simulink model "DCMG_model02"  (R2023a)
settings: Solver=FixedStepDiscrete  StartTime=0.0  StopTime=7  FixedStep=Ts  RelTol=1e-3
InitFcn:
  | Ts=10e-6;
  | R1=0.5;
  | R2=0.6;
  | RD1=4;
  | RD2=4;
  | Vdc1=350;
  | Vdc2=350;
  | Vdcmg_ref=125;
  | Vc1_ref=125;
  | Vc2_ref=125;
libraries: spsSeriesRLCBranchLib x7, spsCurrentMeasurementLib x5, slpidlib x5, spsVoltageMeasurementLib x3, spsDiodeLib x3, spsMosfetLib x3, spsControlledCurrentSourceLib x2, spsDCVoltageSourceLib x2, spsGroundLib x1, spsThreePhaseBreakerLib x1, sps_lib x1
settings Model: Creator=Aminsystem  LastModifiedBy=Aminsystem
settings DataIOCC: SaveOutput=off  SignalLogging=off  DSMLogging=off  SaveTime=off  ReturnWorkspaceOutputs=off

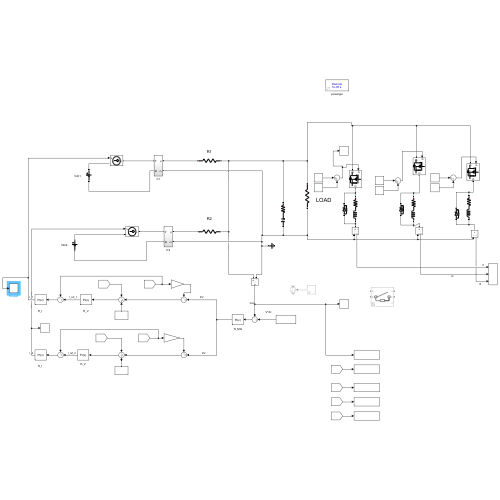
[thumbnail: Simulink's stored preview of the top-level diagram]
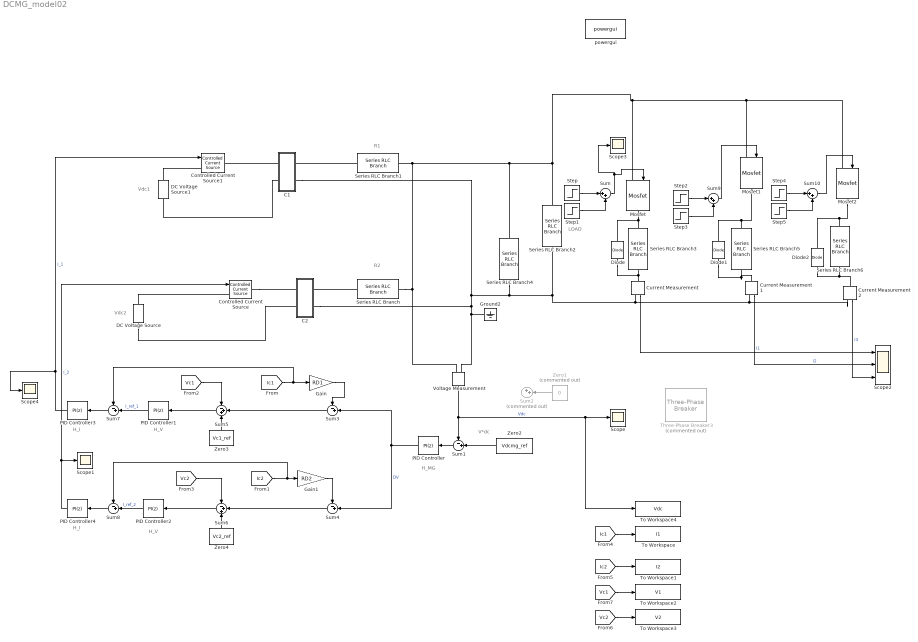
== system DCMG_model02 ==
  note: H_V
  note: Vdc2
  note: Vdc1
  note: R2
  note: V*dc
  note: LOAD
  note: R1
  note: H_V
  note: H_MG
  note: H_I
  note: H_I
  C1 : Subsystem
  C2 : Subsystem
  Controlled Current Source : spsControlledCurrentSourceLib/Controlled Current Source  Initialize=on  Source_Type=DC  Amplitude=0  Phase=0  Frequency=0  Measurements=None
  Controlled Current Source1 : spsControlledCurrentSourceLib/Controlled Current Source  Initialize=on  Source_Type=DC  Amplitude=0  Phase=0  Frequency=0  Measurements=None
  Current Measurement : spsCurrentMeasurementLib/Current Measurement  PhasorSimulation=off  OutputType=Complex  PSBequivalent=0
  Current Measurement1 : spsCurrentMeasurementLib/Current Measurement  PhasorSimulation=off  OutputType=Complex  PSBequivalent=0
  Current Measurement2 : spsCurrentMeasurementLib/Current Measurement  PhasorSimulation=off  OutputType=Complex  PSBequivalent=0
  DC Voltage Source : spsDCVoltageSourceLib/DC Voltage Source  Amplitude=Vdc2  Measurements=None
  DC Voltage Source1 : spsDCVoltageSourceLib/DC Voltage Source  Amplitude=Vdc1  Measurements=None
  Diode : spsDiodeLib/Diode  Ron=0.001  Lon=0  Vf=0.8  IC=0  UseSnubber=0  Rs=500  Cs=250e-9  Measurements=off
  Diode1 : spsDiodeLib/Diode  Ron=0.001  Lon=0  Vf=0.8  IC=0  UseSnubber=0  Rs=500  Cs=250e-9  Measurements=off
  Diode2 : spsDiodeLib/Diode  Ron=0.001  Lon=0  Vf=0.8  IC=0  UseSnubber=0  Rs=500  Cs=250e-9  Measurements=off
  Gain : Gain  Gain=RD1
  Gain1 : Gain  Gain=RD2
  Ground2 : spsGroundLib/Ground  LConnTagsString=a
  Mosfet : spsMosfetLib/Mosfet  Ron=0.1  Lon=0  Rd=0.01  Vfd=0  IC=0  Rs=1e5  Cs=inf  Measurements=off
  Mosfet1 : spsMosfetLib/Mosfet  Ron=0.1  Lon=0  Rd=0.01  Vfd=0  IC=0  Rs=1e5  Cs=inf  Measurements=off
  Mosfet2 : spsMosfetLib/Mosfet  Ron=0.1  Lon=0  Rd=0.01  Vfd=0  IC=0  Rs=1e5  Cs=inf  Measurements=off
  PID Controller{,1..4} (5 alike) : slpidlib/PID Controller  Controller=PI  Form=Parallel  TimeDomain=Discrete-time  UseExternalTs=off  SampleTime=Ts  IntegratorMethod=Forward Euler  FilterMethod=Forward Euler  ControllerParametersSource=internal  P=10  I=100  UseKiTs=off  D=0  N=100  UseFilter=on  TunerSelectOption=Transfer Function Based (PID Tuner App)  InitialConditionSource=internal  InitialConditionForIntegrator=0  InitialConditionForFilter=0  DifferentiatorICPrevScaledInput=0  ExternalReset=none  TrackingMode=off  Kt=1  LimitOutput=off  SatLimitsSource=internal  UpperSaturationLimit=inf  LowerSaturationLimit=-inf  LinearizeAsGain=on  AntiWindupMode=none  Kb=1  LimitIntegrator=off  UpperIntegratorSaturationLimit=inf  LowerIntegratorSaturationLimit=-inf  POutMin=[]  POutMax=[]  IOutMin=[]  IOutMax=[]  DOutMin=[]  DOutMax=[]  NOutMin=[]  NOutMax=[]  SumOutMin=[]  SumOutMax=[]  SaturationOutMin=[]  SaturationOutMax=[]  PParamMin=[]  PParamMax=[]  IParamMin=[]  IParamMax=[]  DParamMin=[]  DParamMax=[]  NParamMin=[]  NParamMax=[]  KbParamMin=[]  KbParamMax=[]  KtParamMin=[]  KtParamMax=[]  KbOutMin=[]  KbOutMax=[]  KtOutMin=[]  KtOutMax=[]  IntegratorOutMin=[]  IntegratorOutMax=[]  FilterOutMin=[]  FilterOutMax=[]  SumI1OutMin=[]  SumI1OutMax=[]  SumI2OutMin=[]  SumI2OutMax=[]  SumI3OutMin=[]  SumI3OutMax=[]  SumI4OutMin=[]  SumI4OutMax=[]  SumDOutMin=[]  SumDOutMax=[]  DifferentiatorOutMin=[]  DifferentiatorOutMax=[]  FilterDiffOutCoefMin=[]  FilterDiffOutCoefMax=[]  ReciprocalOutMin=[]  ReciprocalOutMax=[]  SumDenOutMin=[]  SumDenOutMax=[]  SumNumOutMin=[]  SumNumOutMax=[]  DivideOutMin=[]  DivideOutMax=[]  UdiffTsProdOutMin=[]  UdiffTsProdOutMax=[]  NTsProdOutMin=[]  NTsProdOutMax=[]  UintegralTsProdOutMin=[]  UintegralTsProdOutMax=[]  UngainTsProdOutMin=[]  UngainTsProdOutMax=[]  ClampingZeroOutDataTypeStr=Inherit: Inherit via back propagation  ClampingZeroOutMin=[]  ClampingZeroOutMax=[]  FilterDenConstantOutDataTypeStr=Inherit: Inherit via back propagation  FilterDenConstantOutMin=[]  FilterDenConstantOutMax=[]  PCopyOutDataTypeStr=Inherit: Inherit via back propagation  PCopyOutMin=[]  PCopyOutMax=[]  NCopyOutDataTypeStr=Inherit: Inherit via back propagation  NCopyOutMin=[]  NCopyOutMax=[]  IntegratorContinuousStateAttributes=''  IntegratorStateMustResolveToSignalObject=off  IntegratorRTWStateStorageClass=Auto  FilterContinuousStateAttributes=''  FilterStateMustResolveToSignalObject=off  FilterRTWStateStorageClass=Auto  ParallelPVariant=InternalParameters  IdealPVariant=Disabled  IVariant=InternalParameters  DVariant=Disabled  IntegratorVariant=Discrete  SatVariant=Disabled  AWVariant=Passthrough  PCopyVariant=Disabled  TRVariant=Disabled  FdbkBlocksVariant=Forward  IdealPFdbkVariant=Disabled  SatFdbkVariant=Disabled  DerivativeFilterVariant=Disabled  NVariant=Disabled  NCopyVariant=Disabled_SignalSpec  FilterICVariant=Disabled  IntegratorICVariant=InternalICs  ExternalResetVariant=Disabled  TRSumVariant=Passthrough  SumFdbkVariant=Disabled  SumVariant=Sum_PI  TsampFilterVariant=InternalTs  TsampNgainVariant=Passthrough  TsampIntegralVariant=Disabled_SignalSpec  ExternalSaturationOutDataTypeStr=Inherit: Same as second input
  Scope{,1,3..4} (4 alike) : Scope
  Scope2 : Scope  NumInputPorts=3
  Series RLC Branch : spsSeriesRLCBranchLib/Series RLC Branch  LConnTagsString=__new0  RConnTagsString=__new0  BranchType=R  Resistance=R2  Inductance=1e-3  SetiL0=off  InitialCurrent=0  Capacitance=1e-6  Setx0=off  InitialVoltage=0  Measurements=None
  Series RLC Branch1 : spsSeriesRLCBranchLib/Series RLC Branch  LConnTagsString=__new0  RConnTagsString=__new0  BranchType=R  Resistance=R1  Inductance=1e-3  SetiL0=off  InitialCurrent=0  Capacitance=1e-6  Setx0=off  InitialVoltage=0  Measurements=None
  Series RLC Branch2 : spsSeriesRLCBranchLib/Series RLC Branch  LConnTagsString=__new0  RConnTagsString=__new0  BranchType=R  Resistance=120  Inductance=1e-3  SetiL0=off  InitialCurrent=0  Capacitance=1e-6  Setx0=off  InitialVoltage=0  Measurements=None
  Series RLC Branch3 : spsSeriesRLCBranchLib/Series RLC Branch  LConnTagsString=__new0  RConnTagsString=__new0  BranchType=RL  Resistance=1  Inductance=2e-3  SetiL0=off  InitialCurrent=0  Capacitance=1e-6  Setx0=off  InitialVoltage=0  Measurements=None
  Series RLC Branch4 : spsSeriesRLCBranchLib/Series RLC Branch  LConnTagsString=__new0  RConnTagsString=__new0  BranchType=RC  Resistance=0.1  Inductance=1e-3  SetiL0=off  InitialCurrent=0  Capacitance=100e-6  Setx0=on  InitialVoltage=80  Measurements=None
  Series RLC Branch5 : spsSeriesRLCBranchLib/Series RLC Branch  LConnTagsString=__new0  RConnTagsString=__new0  BranchType=RL  Resistance=0.5  Inductance=5e-3  SetiL0=off  InitialCurrent=0  Capacitance=1e-6  Setx0=off  InitialVoltage=0  Measurements=None
  Series RLC Branch6 : spsSeriesRLCBranchLib/Series RLC Branch  LConnTagsString=__new0  RConnTagsString=__new0  BranchType=RL  Resistance=1  Inductance=10e-3  SetiL0=off  InitialCurrent=0  Capacitance=1e-6  Setx0=off  InitialVoltage=0  Measurements=None
  Step : Step  Time=1.3  SampleTime=Ts
  Step1 : Step  Time=2.3  After=-1  SampleTime=Ts
  Step2 : Step  Time=3  SampleTime=Ts
  Step3 : Step  Time=4  After=-1  SampleTime=Ts
  Step4 : Step  Time=5  SampleTime=Ts
  Step5 : Step  Time=6  After=-1  SampleTime=Ts
  Sum : Sum  Inputs=|++
  Sum{1,3..4,7..8} (5 alike) : Sum  Inputs=-+|
  Sum10 : Sum  Inputs=|++
  Sum2 : Sum  Commented=on  Inputs=|++
  Sum5 : Sum  Inputs=-++
  Sum6 : Sum  Inputs=-++
  Sum9 : Sum  Inputs=|++
  Three-Phase Breaker3 : spsThreePhaseBreakerLib/Three-Phase Breaker  Commented=on  InitialState=open  SwitchA=on  SwitchB=on  SwitchC=on  SwitchTimes="[1/60  5/60]"  External=off  BreakerResistance=0.01  SnubberResistance=1e6  SnubberCapacitance=inf  Measurements=None
  To Workspace : ToWorkspace  VariableName=I1  SaveFormat=Structure With Time  SampleTime=Ts
  To Workspace1 : ToWorkspace  VariableName=I2  SaveFormat=Structure With Time  SampleTime=Ts
  To Workspace2 : ToWorkspace  VariableName=V1  SaveFormat=Structure With Time  SampleTime=Ts
  To Workspace3 : ToWorkspace  VariableName=V2  SaveFormat=Structure With Time  SampleTime=Ts
  To Workspace4 : ToWorkspace  VariableName=Vdc  SaveFormat=Structure With Time  SampleTime=Ts
  Voltage Measurement : spsVoltageMeasurementLib/Voltage Measurement  PhasorSimulation=off  OutputType=Complex  PSBequivalent=0
  Zero1 : Constant  Commented=on  Value=0  OutDataTypeStr=Inherit: Inherit via back propagation
  Zero2 : Constant  Value=Vdcmg_ref  OutDataTypeStr=Inherit: Inherit via back propagation  SampleTime=Ts
  Zero3 : Constant  Value=Vc1_ref  OutDataTypeStr=Inherit: Inherit via back propagation
  Zero4 : Constant  Value=Vc2_ref  OutDataTypeStr=Inherit: Inherit via back propagation
  powergui : sps_lib/powergui  Priority=1  SimulationMode=Discrete  SampleTime=Ts  frequency=60  Iterations=50  frequencyindice=0  Pbase=100e6  ErrMax=1e-4  UnitsV=kV  UnitsW=MW  buscounter=0  FunctionMessages=off  echomessages=off  EnableUseOfTLC=off  CurrentSourceSwitches=off  DisableSnubberDevices=off  DisableRonSwitches=off  DisableVfSwitches=off  DisplayEquations=off  AutomaticDiscreteSolvers=off  SolverType=Tustin/Backward Euler (TBE)  Interpol=off  ExternalGateDelay=off  methode=off  Ts=100  x0status=blocks  SPID=on  SwTol=0  HookPort=off  NonlinearTolerance=1e-4  nMaxIteration=100  ContinueOnMaxIteration=off  RestoreLinks=warning  ResistiveCurrentMeasurement=off  Frange=[0:2:500]  Ylog=off  Xlog=on  ShowGrid=off  save=off  variable=ZData  structure=0  ZoomFFT=off  StartTime=0.0  cycles=1  DisplayStyle=1  fundamental=60  FreqAxis=off  MaxFrequency=1000  frequencyindicesteady=1  RmsSteady=1  display=off
  wires:
  Voltage Measurement/1 -> To Workspace4/1, Scope/1, Sum1/1  "Vdc"
  Zero1/1 -> Sum2/2
  Zero2/1 -> Sum1/2
  Sum1/1 -> PID Controller/1
  PID Controller/1 -> Sum4/2, Sum3/2  "DV"
  [Ic1] -> Sum7/1, Gain/1
  Gain/1 -> Sum3/1
  [Ic2] -> Sum8/1, Gain1/1
  Gain1/1 -> Sum4/1
  Sum3/1 -> Sum5/2
  Zero3/1 -> Sum5/3
  Zero4/1 -> Sum6/3
  Sum4/1 -> Sum6/2
  [Vc1] -> Sum5/1
  [Vc2] -> Sum6/1
  Sum5/1 -> PID Controller1/1
  Sum6/1 -> PID Controller2/1
  PID Controller1/1 -> Sum7/2  "I_ref_1"
  PID Controller2/1 -> Sum8/2  "I_ref_2"
  Sum7/1 -> PID Controller3/1
  Sum8/1 -> PID Controller4/1
  PID Controller3/1 -> Controlled Current Source1/1, Scope4/1  "I_1"
  PID Controller4/1 -> Controlled Current Source/1, Scope1/1  "I_2"
  Step/1 -> Sum/1
  Step1/1 -> Sum/2
  Sum/1 -> Mosfet/1, Scope3/1
  Step3/1 -> Sum9/2
  Step2/1 -> Sum9/1
  Step4/1 -> Sum10/1
  Step5/1 -> Sum10/2
  Current Measurement/1 -> Scope2/1  "I1"
  Current Measurement1/1 -> Scope2/2  "I2"
  Current Measurement2/1 -> Scope2/3  "I3"
  Sum9/1 -> Mosfet1/1
  Sum10/1 -> Mosfet2/1
  [Ic1] -> To Workspace/1
  [Ic2] -> To Workspace1/1
  [Vc1] -> To Workspace2/1
  [Vc2] -> To Workspace3/1
  connections:
  DC Voltage Source/LConn1 -- C2/LConn2
  Controlled Current Source1/LConn1 -- DC Voltage Source1/RConn1
  C1/LConn2 -- DC Voltage Source1/LConn1
  C1/LConn1 -- Controlled Current Source1/RConn1
  Series RLC Branch5/RConn1 -- Diode1/LConn1 -- Current Measurement1/LConn1
  Series RLC Branch2/LConn1 -- Mosfet2/LConn1 -- Mosfet1/LConn1 -- Mosfet/LConn1 -- Series RLC Branch/RConn1 -- Voltage Measurement/LConn1 -- Series RLC Branch1/RConn1 -- Series RLC Branch4/LConn1
  Series RLC Branch/LConn1 -- C2/RConn1
  Series RLC Branch1/LConn1 -- C1/RConn1
  Mosfet/RConn1 -- Diode/RConn1 -- Series RLC Branch3/LConn1
  Controlled Current Source/RConn1 -- C2/LConn1
  Controlled Current Source/LConn1 -- DC Voltage Source/RConn1
  Series RLC Branch3/RConn1 -- Diode/LConn1 -- Current Measurement/LConn1
  Voltage Measurement/LConn2 -- C2/RConn2 -- C1/RConn2 -- Current Measurement2/RConn1 -- Current Measurement1/RConn1 -- Current Measurement/RConn1 -- Series RLC Branch2/RConn1 -- Series RLC Branch4/RConn1 -- Ground2/LConn1
  Current Measurement2/LConn1 -- Diode2/LConn1 -- Series RLC Branch6/RConn1
  Series RLC Branch5/LConn1 -- Mosfet1/RConn1 -- Diode1/RConn1
  Diode2/RConn1 -- Mosfet2/RConn1 -- Series RLC Branch6/LConn1

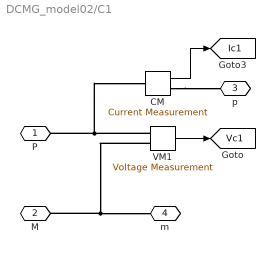
== system DCMG_model02/C1 ==
  CM : spsCurrentMeasurementLib/Current Measurement  PhasorSimulation=off  OutputType=Complex  PSBequivalent=0
  VM1 : spsVoltageMeasurementLib/Voltage Measurement  PhasorSimulation=off  OutputType=Complex  PSBequivalent=0
  P : PMIOPort  Side=Left
  M : PMIOPort  Port=2  Side=Left
  p : PMIOPort  Port=3  Side=Right
  m : PMIOPort  Port=4  Side=Right
  tag scope: Ic1=global, Vc1=global
  wires:
  VM1/1 -> [Vc1]
  CM/1 -> [Ic1]
  connections:
  P/RConn1 -- VM1/LConn1 -- CM/LConn1
  M/RConn1 -- VM1/LConn2 -- m/RConn1
  CM/RConn1 -- p/RConn1

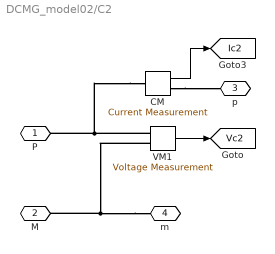
== system DCMG_model02/C2 ==
  CM : spsCurrentMeasurementLib/Current Measurement  PhasorSimulation=off  OutputType=Complex  PSBequivalent=0
  VM1 : spsVoltageMeasurementLib/Voltage Measurement  PhasorSimulation=off  OutputType=Complex  PSBequivalent=0
  P : PMIOPort  Side=Left
  M : PMIOPort  Port=2  Side=Left
  p : PMIOPort  Port=3  Side=Right
  m : PMIOPort  Port=4  Side=Right
  tag scope: Ic2=global, Vc2=global
  wires:
  CM/1 -> [Ic2]
  VM1/1 -> [Vc2]
  connections:
  CM/RConn1 -- p/RConn1
  m/RConn1 -- VM1/LConn2 -- M/RConn1
  CM/LConn1 -- VM1/LConn1 -- P/RConn1
